simulink model "Scenario_3_v2"  (R2020b)
settings: Solver=ode1be  StartTime=0.0  StopTime=0.5  FixedStep=Ts  MaxStep=Ts/10  MinStep=Ts/40  RelTol=1e-3
values from neighbouring files (symbols this model uses):
  c0 = c0_zeb    (= 6.57988e-09)    [Scenario_17_parameters_v2.m]    (also in Scenario_1_parameters_v2.m; Scenario_2_parameters_v2.m; Scenario_3_parameters_v2.m)
  c0_hawk = 6.37282e-09    [Scenario_17_parameters_v2.m]    (also in Scenario_1_parameters_v2.m; Scenario_2_parameters_v2.m; Scenario_3_parameters_v2.m)
  c1 = c1_zeb    (= 9.15905e-09)    [Scenario_17_parameters_v2.m]    (also in Scenario_1_parameters_v2.m; Scenario_2_parameters_v2.m; Scenario_3_parameters_v2.m)
  c1_hawk = 8.76156e-09    [Scenario_17_parameters_v2.m]    (also in Scenario_1_parameters_v2.m; Scenario_2_parameters_v2.m; Scenario_3_parameters_v2.m)
  fg = 50    [Scenario_17_parameters_v2.m]    (also in Scenario_1_parameters_v2.m; Scenario_2_parameters_v2.m; Scenario_3_parameters_v2.m)
  G10gen = 0.90    (= 0.9)    [Scenario_3_parameters_v2.m]
  G12gen = 0.85    [Scenario_3_parameters_v2.m]
  G1gen = 0.4692    [Scenario_17_parameters_v2.m]    (also in Scenario_1_parameters_v2.m = 0.1; Scenario_2_parameters_v2.m = 0.298581; Scenario_3_parameters_v2.m = 0.65)
  G2gen = 0.80    (= 0.8)    [Scenario_1_parameters_v2.m]    (also in Scenario_2_parameters_v2.m = 0.7; Scenario_3_parameters_v2.m = 0.4)
  G3gen = 0.85    [Scenario_1_parameters_v2.m]    (also in Scenario_2_parameters_v2.m = 0.9; Scenario_3_parameters_v2.m = 0.6)
  G4gen = 0.65    [Scenario_3_parameters_v2.m]
  G5gen = 0.75    [Scenario_17_parameters_v2.m]    (also in Scenario_1_parameters_v2.m = 0.8; Scenario_2_parameters_v2.m = 0.8; Scenario_3_parameters_v2.m = 0.705)
  G6gen = 0.90    (= 0.9)    [Scenario_17_parameters_v2.m]    (also in Scenario_1_parameters_v2.m; Scenario_2_parameters_v2.m = 0.81797; Scenario_3_parameters_v2.m = 0.45)
  G7gen = 0.20    (= 0.2)    [Scenario_17_parameters_v2.m]    (also in Scenario_1_parameters_v2.m = 0.5227; Scenario_2_parameters_v2.m = 0.5098; Scenario_3_parameters_v2.m = 0.4)
  G8gen = 0.58    [Scenario_17_parameters_v2.m]    (also in Scenario_3_parameters_v2.m = 0.65)
  G9gen = 0.8833    [Scenario_17_parameters_v2.m]    (also in Scenario_3_parameters_v2.m = 0.9)
  Iovc = 1.2    [Scenario_17_parameters_v2.m]    (also in Scenario_1_parameters_v2.m; Scenario_2_parameters_v2.m; Scenario_3_parameters_v2.m)
  l0 = l0_zeb    (= 0.00368)    [Scenario_17_parameters_v2.m]    (also in Scenario_1_parameters_v2.m; Scenario_2_parameters_v2.m; Scenario_3_parameters_v2.m)
  l0_hawk = 0.00373    [Scenario_17_parameters_v2.m]    (also in Scenario_1_parameters_v2.m; Scenario_2_parameters_v2.m; Scenario_3_parameters_v2.m)
  l1 = l1_zeb    (= 0.00128)    [Scenario_17_parameters_v2.m]    (also in Scenario_1_parameters_v2.m; Scenario_2_parameters_v2.m; Scenario_3_parameters_v2.m)
  L10dem = 0.04    [Scenario_3_parameters_v2.m]
  L12dem = 0.01    [Scenario_17_parameters_v2.m]    (also in Scenario_3_parameters_v2.m = 0.02)
  L13dem = 0.01    [Scenario_3_parameters_v2.m]
  l1_hawk = 0.00133    [Scenario_17_parameters_v2.m]    (also in Scenario_1_parameters_v2.m; Scenario_2_parameters_v2.m; Scenario_3_parameters_v2.m)
  L1dem = 0.25    [Scenario_17_parameters_v2.m]    (also in Scenario_3_parameters_v2.m = 0.1)
  L3dem = 0.30    (= 0.3)    [Scenario_17_parameters_v2.m]    (also in Scenario_1_parameters_v2.m = 0.1; Scenario_2_parameters_v2.m = 0.1; Scenario_3_parameters_v2.m = 0.2)
  L5dem = 0.25    [Scenario_17_parameters_v2.m]    (also in Scenario_1_parameters_v2.m = 0.35; Scenario_2_parameters_v2.m = 0.35; Scenario_3_parameters_v2.m = 0.1)
  L6dem = 0.15    [Scenario_1_parameters_v2.m]    (also in Scenario_2_parameters_v2.m; Scenario_3_parameters_v2.m = 0.1)
  L7dem = 0.10    (= 0.1)    [Scenario_1_parameters_v2.m]    (also in Scenario_2_parameters_v2.m; Scenario_3_parameters_v2.m = 0.2)
  L9dem = 0.15    [Scenario_17_parameters_v2.m]    (also in Scenario_3_parameters_v2.m = 0.1)
  Pr = Sr*PF    (= 1600500000)    [Scenario_17_parameters_v2.m]    (also in Scenario_1_parameters_v2.m = 1472500000; Scenario_2_parameters_v2.m = 1805000000; Scenario_3_parameters_v2.m = 12740000000)
  Qr = sqrt(Sr^2 - Pr^2)    [Scenario_17_parameters_v2.m]    (also in Scenario_1_parameters_v2.m; Scenario_2_parameters_v2.m; Scenario_3_parameters_v2.m)
  r0 = r0_zeb    (= 0.39362)    [Scenario_17_parameters_v2.m]    (also in Scenario_1_parameters_v2.m; Scenario_2_parameters_v2.m; Scenario_3_parameters_v2.m)
  r0_hawk = 0.44587    [Scenario_17_parameters_v2.m]    (also in Scenario_1_parameters_v2.m; Scenario_2_parameters_v2.m; Scenario_3_parameters_v2.m)
  r1 = r1_zeb    (= 0.06862)    [Scenario_17_parameters_v2.m]    (also in Scenario_1_parameters_v2.m; Scenario_2_parameters_v2.m; Scenario_3_parameters_v2.m)
  r1_hawk = 0.12087    [Scenario_17_parameters_v2.m]    (also in Scenario_1_parameters_v2.m; Scenario_2_parameters_v2.m; Scenario_3_parameters_v2.m)
  Rtpu = Xtpu/40    (= 0.0025)    [Scenario_17_parameters_v2.m]    (also in Scenario_1_parameters_v2.m = 0.00375; Scenario_2_parameters_v2.m = 0.00375; Scenario_3_parameters_v2.m)
  S10non = 500e6    (= 500000000)    [Scenario_3_parameters_v2.m]
  S12non = 250e6    (= 250000000)    [Scenario_3_parameters_v2.m]
  S1non = 700e6    (= 700000000)    [Scenario_17_parameters_v2.m]    (also in Scenario_1_parameters_v2.m = 400000000; Scenario_2_parameters_v2.m = 400000000; Scenario_3_parameters_v2.m = 1000000000)
  S2non = 300e6    (= 300000000)    [Scenario_1_parameters_v2.m]    (also in Scenario_2_parameters_v2.m; Scenario_3_parameters_v2.m = 3000000000)
  S3non = 200e6    (= 200000000)    [Scenario_1_parameters_v2.m]    (also in Scenario_2_parameters_v2.m; Scenario_3_parameters_v2.m = 1000000000)
  S4non = 2000e6    (= 2000000000)    [Scenario_3_parameters_v2.m]
  S5non = 400e6    (= 400000000)    [Scenario_17_parameters_v2.m]    (also in Scenario_1_parameters_v2.m = 500000000; Scenario_2_parameters_v2.m = 500000000; Scenario_3_parameters_v2.m = 2000000000)
  S6non = 150e6    (= 150000000)    [Scenario_17_parameters_v2.m]    (also in Scenario_1_parameters_v2.m = 400000000; Scenario_2_parameters_v2.m = 400000000; Scenario_3_parameters_v2.m = 3000000000)
  S7non = 1500e6    (= 1500000000)    [Scenario_17_parameters_v2.m]    (also in Scenario_1_parameters_v2.m = 200000000; Scenario_2_parameters_v2.m = 200000000; Scenario_3_parameters_v2.m = 4000000000)
  S8non = 600e6    (= 600000000)    [Scenario_17_parameters_v2.m]    (also in Scenario_3_parameters_v2.m = 2000000000)
  S9non = 200e6    (= 200000000)    [Scenario_17_parameters_v2.m]    (also in Scenario_3_parameters_v2.m = 1500000000)
  tonvsc = 0    [Scenario_17_parameters_v2.m]    (also in Scenario_1_parameters_v2.m; Scenario_2_parameters_v2.m; Scenario_3_parameters_v2.m = 0.0001)
  Ts = 50e-6    (= 5e-05)    [Scenario_17_parameters_v2.m]    (also in Scenario_1_parameters_v2.m = 0.0002; Scenario_2_parameters_v2.m = 2e-05; Scenario_3_parameters_v2.m = 0.0001)
  Vhv = 220e3    (= 220000)    [Scenario_17_parameters_v2.m]    (also in Scenario_1_parameters_v2.m; Scenario_2_parameters_v2.m; Scenario_3_parameters_v2.m)
  Vmv = 22e3    (= 22000)    [Scenario_17_parameters_v2.m]    (also in Scenario_1_parameters_v2.m; Scenario_2_parameters_v2.m; Scenario_3_parameters_v2.m)
  w_pll = 2*pi*80    (= 502.654824574)    [Scenario_17_parameters_v2.m]    (also in Scenario_1_parameters_v2.m; Scenario_2_parameters_v2.m; Scenario_3_parameters_v2.m)
  wc1 = wsw1/10    (= 848.230016469)    [Scenario_17_parameters_v2.m]    (also in Scenario_1_parameters_v2.m; Scenario_2_parameters_v2.m; Scenario_3_parameters_v2.m)
  wdc1 = wc1/10    (= 84.8230016469)    [Scenario_17_parameters_v2.m]    (also in Scenario_1_parameters_v2.m; Scenario_2_parameters_v2.m; Scenario_3_parameters_v2.m)
  wpq1 = wc1/10    (= 84.8230016469)    [Scenario_17_parameters_v2.m]    (also in Scenario_1_parameters_v2.m; Scenario_2_parameters_v2.m; Scenario_3_parameters_v2.m)
  wsw1 = ksw1*2*pi*fg    (= 8482.30016469)    [Scenario_17_parameters_v2.m]    (also in Scenario_1_parameters_v2.m; Scenario_2_parameters_v2.m; Scenario_3_parameters_v2.m)
  Xtpu = 0.10    (= 0.1)    [Scenario_17_parameters_v2.m]    (also in Scenario_1_parameters_v2.m = 0.15; Scenario_2_parameters_v2.m = 0.15; Scenario_3_parameters_v2.m)
undefined symbols (not defined in the file or in its folder): D11, Delta
libraries: powerlib x428, simulink_extras x272, powerlib_meascontrol x194, pid_lib x105, simulink x60, eeTransforms x54, spsFirstOrderFilterLib x36, eePwmGeneratorTwoLevel x9
(part 34 of 40)

== system Scenario_3_v2/HVDC/VSC1 v2/VSC Control/Control loops/Phasor PQ 1st/Outer-loop ==
  note: Limits the converter current
  note: Frequency droop
  note: Voltage droop
  note: Reactive power control
  note: Active power control
  note: LVRT
  Pset : Inport
  Qset : Inport  Port=2
  vqd+- : Inport  Port=3
  iqd+- : Inport  Port=4
  freq : Inport  Port=5
  Blk : Inport  Port=6
  Cartesian to Polar : simulink_extras/Transformations/Cartesian to Polar
  Compare To Constant1 : simulink/Logic and Bit Operations/Compare To Constant  relop=<  const=0  OutDataTypeStr=boolean
  Constant1 : Constant  Value=fg
  Constant10 : Constant  Value=0
  Constant11 : Constant  Value=Vlvrt0
  Constant2 : Constant  Value=Vmvpk
  Constant9 : Constant  Value=0
  Demux1 : Demux
  Demux2 : Demux
  Divide1 : Product  Inputs=*/
  Divide2 : Product  Inputs=*/
  First-Order Filter : powerlib_meascontrol/Filters/First-Order Filter  FilterType=Lowpass  Tc=1/wpq  Ts=0  Initialize=on  Vac_Init=[0, 0, 60]  Vdc_Init=Icq  PlotResponse=off  FreqRange="[0,  200,  1]"
  First-Order Filter1 : powerlib_meascontrol/Filters/First-Order Filter  FilterType=Lowpass  Tc=2e-3  Ts=0  Initialize=on  Vac_Init=[0, 0, 60]  Vdc_Init=Vgq  PlotResponse=off  FreqRange="[0,  200,  1]"
  First-Order Filter2 : powerlib_meascontrol/Filters/First-Order Filter  FilterType=Lowpass  Tc=1/wpq  Ts=0  Initialize=on  Vac_Init=[0, 0, 60]  Vdc_Init=Icd  PlotResponse=off  FreqRange="[0,  200,  1]"
  First-Order Filter3 : powerlib_meascontrol/Filters/First-Order Filter  FilterType=Lowpass  Tc=20e-3  Ts=0  Initialize=on  Vac_Init=[0, 0, 60]  Vdc_Init=fg  PlotResponse=off  FreqRange="[0,  200,  1]"
  Gain : Gain  Gain=2/3
  Gain1 : Gain  Gain=2/3
  Gain14 : Gain  Gain=1/Vmvpk
  Gain15 : Gain  Gain=Klvrt
  Gain16 : Gain  Gain=Iconvbase
  Gain5 : Gain  Gain=1/Kfdroop*(Pconv/fg) * fdroop_en
  Gain6 : Gain  Gain=1/Kvdroop*(Pconv/Vmvpk) * Vacdroop_en
  Mux1 : Mux  Inputs=10
  Polar to Cartesian : simulink_extras/Transformations/Polar to Cartesian
      settings: SourceProductBaseCode=SL
  Power calculation : Subsystem
  Saturation : Saturate  UpperLimit=Imax  LowerLimit=0
  Saturation1 : Saturate  UpperLimit=fdroop_per*Pconv  LowerLimit=-fdroop_per*Pconv
  Saturation2 : Saturate  UpperLimit=Vacdroop_per*Pconv  LowerLimit=-Vacdroop_per*Pconv
  Saturation3 : Saturate  UpperLimit=inf  LowerLimit=eps
  Saturation4 : Saturate  UpperLimit=inf  LowerLimit=eps
  Saturation7 : Saturate  UpperLimit=0  LowerLimit=-Qmax_lvrt
  Step : Step  Commented=on  Time=0.1  After=0.3*3711  SampleTime=0
  Step1 : Step  Commented=on  Time=0.2  After=0.2*3711  SampleTime=0
  Sum11 : Sum  Inputs=|+-
  Sum3 : Sum  Inputs=|++
  Sum4 : Sum  Inputs=|+-
  Sum5 : Sum  Inputs=|++
  Sum6 : Sum  Inputs=|+-
  Switch2 : Switch  Threshold=1
  Terminator : Terminator
  iq+* : Outport
  id+* : Outport  Port=2
  iq-* : Outport  Port=3
  id-* : Outport  Port=4
  m : Outport  Port=5
  wires:
  [vqp] -> Saturation4/1
  Saturation4/1 -> Divide2/2
  Divide2/1 -> Gain1/1
  Gain1/1 -> First-Order Filter2/1
  Gain/1 -> First-Order Filter/1
  [vqp] -> Saturation3/1
  Divide1/1 -> Gain/1
  Saturation3/1 -> Divide1/2
  Constant10/1 -> id-*/1
  Constant9/1 -> iq-*/1
  First-Order Filter3/1 -> Sum4/2
  [f] -> First-Order Filter3/1
  Saturation2/1 -> Sum5/2
  Qset/1 -> Sum5/1
  Cartesian to Polar/2 -> Polar to Cartesian/2
  Polar to Cartesian/1 -> iq+*/1
  Polar to Cartesian/2 -> id+*/1
  Cartesian to Polar/1 -> Saturation/1
  Saturation/1 -> Polar to Cartesian/1
  Sum3/1 -> Divide1/1  "Pref"
  Constant1/1 -> Sum4/1
  Sum4/1 -> Gain5/1
  Saturation1/1 -> Sum3/2
  Sum5/1 -> Divide2/1  "Qref"
  Sum6/1 -> Gain6/1
  [vqfilt] -> Sum6/2
  Constant2/1 -> Sum6/1
  Pset/1 -> Sum3/1
  First-Order Filter/1 -> Cartesian to Polar/1
  Blk/1 -> Terminator/1
  freq/1 -> [f]
  [vqp] -> Mux1/1
  Mux1/1 -> m/1
  First-Order Filter1/1 -> [vqfilt]
  vqd+-/1 -> Demux1/1
  iqd+-/1 -> Demux2/1
  Demux1/1 -> First-Order Filter1/1, [vqp]
  Demux1/2 -> [vdp]
  Demux1/3 -> [vqn]
  Demux1/4 -> [vdn]
  Demux2/1 -> [iqp]
  Demux2/2 -> [idp]
  Demux2/3 -> [iqn]
  Demux2/4 -> [idn]
  [vqp] -> Power calculation/1(vq+)
  [iqp] -> Power calculation/3(iq+)
  Power calculation/1(PQ) -> [PQdq]
  [idp] -> Power calculation/4(id+)
  [vdp] -> Power calculation/2(vd+)
  [vqn] -> Power calculation/5(vq-)
  [vdn] -> Power calculation/6(vd-)
  [iqn] -> Power calculation/7(iq-)
  [idn] -> Power calculation/8(id-)
  [LVRT_true] -> Switch2/2
  First-Order Filter2/1 -> Switch2/3
  Switch2/1 -> Cartesian to Polar/2
  Compare To Constant1/1 -> [LVRT_true]
  Gain16/1 -> Switch2/1
  Gain15/1 -> Saturation7/1
  Saturation7/1 -> Compare To Constant1/1, Gain16/1
  [vqfilt] -> Gain14/1
  Sum11/1 -> Gain15/1
  Gain14/1 -> Sum11/2
  Constant11/1 -> Sum11/1
  [vdp] -> Mux1/2
  [vqn] -> Mux1/3
  [vdn] -> Mux1/4
  [iqn] -> Mux1/7
  [idn] -> Mux1/8
  [f] -> Mux1/9
  [PQdq] -> Mux1/10
  [idp] -> Mux1/6
  [iqp] -> Mux1/5
  Gain5/1 -> Saturation1/1
  Gain6/1 -> Saturation2/1

== system Scenario_3_v2/HVDC/VSC1 v2/VSC Control/Control loops/SW, EMT AVG, Phasor Quasi-EMT/Inner-loop ==
  note: Positive-sequence current control
  note: Negative-sequence current control
  iq+* : Inport
  id+* : Inport  Port=2
  iq-* : Inport  Port=3
  id-* : Inport  Port=4
  Blk : Inport  Port=5
  vqd+- : Inport  Port=6
  iqd+- : Inport  Port=7
  Demux1 : Demux
  Demux2 : Demux
  Gain{,1..3} (4 alike) : Gain  Gain=Xt
  NOT{,1..3} (4 alike) : Logic  Operator=NOT  IconShape=distinctive  AllPortsSameDT=off  OutDataTypeStr=boolean
  PID Controller1 : pid_lib/PID Controller  Controller=PI  Form=Ideal  TimeDomain=Continuous-time  UseExternalTs=off  SampleTime=-1  IntegratorMethod=Forward Euler  FilterMethod=Forward Euler  ControllerParametersSource=internal  P=kp_c  I=1/ti_c  D=0  UseFilter=on  N=100  TunerSelectOption=Transfer Function Based (PID Tuner App)  InitialConditionSource=internal  InitialConditionForIntegrator=0  InitialConditionForFilter=0  DifferentiatorICPrevScaledInput=0  ExternalReset=level  TrackingMode=off  Kt=1  LimitOutput=off  SatLimitsSource=internal  UpperSaturationLimit=10*Vmvpk  LowerSaturationLimit=-10*Vmvpk  LinearizeAsGain=off  AntiWindupMode=none  Kb=1  POutMin=[]  POutMax=[]  IOutMin=[]  IOutMax=[]  DOutMin=[]  DOutMax=[]  NOutMin=[]  NOutMax=[]  SumOutMin=[]  SumOutMax=[]  SaturationOutMin=[]  SaturationOutMax=[]  PParamMin=[]  PParamMax=[]  IParamMin=[]  IParamMax=[]  DParamMin=[]  DParamMax=[]  NParamMin=[]  NParamMax=[]  KbParamMin=[]  KbParamMax=[]  KtParamMin=[]  KtParamMax=[]  KbOutMin=[]  KbOutMax=[]  KtOutMin=[]  KtOutMax=[]  IntegratorOutMin=[]  IntegratorOutMax=[]  FilterOutMin=[]  FilterOutMax=[]  SumI1OutMin=[]  SumI1OutMax=[]  SumI2OutMin=[]  SumI2OutMax=[]  SumI3OutMin=[]  SumI3OutMax=[]  SumI4OutMin=[]  SumI4OutMax=[]  SumDOutMin=[]  SumDOutMax=[]  DifferentiatorOutMin=[]  DifferentiatorOutMax=[]  FilterDiffOutCoefMin=[]  FilterDiffOutCoefMax=[]  ReciprocalOutMin=[]  ReciprocalOutMax=[]  SumDenOutMin=[]  SumDenOutMax=[]  SumNumOutMin=[]  SumNumOutMax=[]  DivideOutMin=[]  DivideOutMax=[]  UdiffTsProdOutMin=[]  UdiffTsProdOutMax=[]  NTsProdOutMin=[]  NTsProdOutMax=[]  UintegralTsProdOutMin=[]  UintegralTsProdOutMax=[]  UngainTsProdOutMin=[]  UngainTsProdOutMax=[]  IntegratorContinuousStateAttributes=''  IntegratorStateMustResolveToSignalObject=off  IntegratorRTWStateStorageClass=Auto  FilterContinuousStateAttributes=''  FilterStateMustResolveToSignalObject=off  FilterRTWStateStorageClass=Auto  ParallelPVariant=Passthrough  IdealPVariant=InternalParameters  IVariant=InternalParameters  DVariant=Disabled  IntegratorVariant=Continuous  SatVariant=Disabled  AWVariant=Passthrough  PCopyVariant=Disabled  TRVariant=Disabled  FdbkBlocksVariant=Forward  IdealPFdbkVariant=Disabled  SatFdbkVariant=Disabled  DerivativeFilterVariant=Disabled  NVariant=Disabled  NCopyVariant=Disabled_SignalSpec  FilterICVariant=Disabled  IntegratorICVariant=InternalICs  ExternalResetVariant=ExternalReset  TRSumVariant=Passthrough  SumFdbkVariant=Disabled  SumVariant=Sum_PI  TsampFilterVariant=InternalTs  TsampNgainVariant=Passthrough  TsampIntegralVariant=Passthrough  ExternalSaturationOutDataTypeStr=Inherit: Same as second input
  PID Controller2 : pid_lib/PID Controller  Controller=PI  Form=Ideal  TimeDomain=Continuous-time  UseExternalTs=off  SampleTime=-1  IntegratorMethod=Forward Euler  FilterMethod=Forward Euler  ControllerParametersSource=internal  P=kp_c  I=1/ti_c  D=0  UseFilter=on  N=100  TunerSelectOption=Transfer Function Based (PID Tuner App)  InitialConditionSource=internal  InitialConditionForIntegrator=Tcq/kp_c  InitialConditionForFilter=0  DifferentiatorICPrevScaledInput=0  ExternalReset=level  TrackingMode=off  Kt=1  LimitOutput=off  SatLimitsSource=internal  UpperSaturationLimit=10*Vmvpk  LowerSaturationLimit=-10*Vmvpk  LinearizeAsGain=off  AntiWindupMode=none  Kb=1  POutMin=[]  POutMax=[]  IOutMin=[]  IOutMax=[]  DOutMin=[]  DOutMax=[]  NOutMin=[]  NOutMax=[]  SumOutMin=[]  SumOutMax=[]  SaturationOutMin=[]  SaturationOutMax=[]  PParamMin=[]  PParamMax=[]  IParamMin=[]  IParamMax=[]  DParamMin=[]  DParamMax=[]  NParamMin=[]  NParamMax=[]  KbParamMin=[]  KbParamMax=[]  KtParamMin=[]  KtParamMax=[]  KbOutMin=[]  KbOutMax=[]  KtOutMin=[]  KtOutMax=[]  IntegratorOutMin=[]  IntegratorOutMax=[]  FilterOutMin=[]  FilterOutMax=[]  SumI1OutMin=[]  SumI1OutMax=[]  SumI2OutMin=[]  SumI2OutMax=[]  SumI3OutMin=[]  SumI3OutMax=[]  SumI4OutMin=[]  SumI4OutMax=[]  SumDOutMin=[]  SumDOutMax=[]  DifferentiatorOutMin=[]  DifferentiatorOutMax=[]  FilterDiffOutCoefMin=[]  FilterDiffOutCoefMax=[]  ReciprocalOutMin=[]  ReciprocalOutMax=[]  SumDenOutMin=[]  SumDenOutMax=[]  SumNumOutMin=[]  SumNumOutMax=[]  DivideOutMin=[]  DivideOutMax=[]  UdiffTsProdOutMin=[]  UdiffTsProdOutMax=[]  NTsProdOutMin=[]  NTsProdOutMax=[]  UintegralTsProdOutMin=[]  UintegralTsProdOutMax=[]  UngainTsProdOutMin=[]  UngainTsProdOutMax=[]  IntegratorContinuousStateAttributes=''  IntegratorStateMustResolveToSignalObject=off  IntegratorRTWStateStorageClass=Auto  FilterContinuousStateAttributes=''  FilterStateMustResolveToSignalObject=off  FilterRTWStateStorageClass=Auto  ParallelPVariant=Passthrough  IdealPVariant=InternalParameters  IVariant=InternalParameters  DVariant=Disabled  IntegratorVariant=Continuous  SatVariant=Disabled  AWVariant=Passthrough  PCopyVariant=Disabled  TRVariant=Disabled  FdbkBlocksVariant=Forward  IdealPFdbkVariant=Disabled  SatFdbkVariant=Disabled  DerivativeFilterVariant=Disabled  NVariant=Disabled  NCopyVariant=Disabled_SignalSpec  FilterICVariant=Disabled  IntegratorICVariant=InternalICs  ExternalResetVariant=ExternalReset  TRSumVariant=Passthrough  SumFdbkVariant=Disabled  SumVariant=Sum_PI  TsampFilterVariant=InternalTs  TsampNgainVariant=Passthrough  TsampIntegralVariant=Passthrough  ExternalSaturationOutDataTypeStr=Inherit: Same as second input
  PID Controller3 : pid_lib/PID Controller  Controller=PI  Form=Ideal  TimeDomain=Continuous-time  UseExternalTs=off  SampleTime=-1  IntegratorMethod=Forward Euler  FilterMethod=Forward Euler  ControllerParametersSource=internal  P=kp_c  I=1/ti_c  D=0  UseFilter=on  N=100  TunerSelectOption=Transfer Function Based (PID Tuner App)  InitialConditionSource=internal  InitialConditionForIntegrator=Tcd/kp_c  InitialConditionForFilter=0  DifferentiatorICPrevScaledInput=0  ExternalReset=level  TrackingMode=off  Kt=1  LimitOutput=off  SatLimitsSource=internal  UpperSaturationLimit=10*Vmvpk  LowerSaturationLimit=-10*Vmvpk  LinearizeAsGain=off  AntiWindupMode=none  Kb=1  POutMin=[]  POutMax=[]  IOutMin=[]  IOutMax=[]  DOutMin=[]  DOutMax=[]  NOutMin=[]  NOutMax=[]  SumOutMin=[]  SumOutMax=[]  SaturationOutMin=[]  SaturationOutMax=[]  PParamMin=[]  PParamMax=[]  IParamMin=[]  IParamMax=[]  DParamMin=[]  DParamMax=[]  NParamMin=[]  NParamMax=[]  KbParamMin=[]  KbParamMax=[]  KtParamMin=[]  KtParamMax=[]  KbOutMin=[]  KbOutMax=[]  KtOutMin=[]  KtOutMax=[]  IntegratorOutMin=[]  IntegratorOutMax=[]  FilterOutMin=[]  FilterOutMax=[]  SumI1OutMin=[]  SumI1OutMax=[]  SumI2OutMin=[]  SumI2OutMax=[]  SumI3OutMin=[]  SumI3OutMax=[]  SumI4OutMin=[]  SumI4OutMax=[]  SumDOutMin=[]  SumDOutMax=[]  DifferentiatorOutMin=[]  DifferentiatorOutMax=[]  FilterDiffOutCoefMin=[]  FilterDiffOutCoefMax=[]  ReciprocalOutMin=[]  ReciprocalOutMax=[]  SumDenOutMin=[]  SumDenOutMax=[]  SumNumOutMin=[]  SumNumOutMax=[]  DivideOutMin=[]  DivideOutMax=[]  UdiffTsProdOutMin=[]  UdiffTsProdOutMax=[]  NTsProdOutMin=[]  NTsProdOutMax=[]  UintegralTsProdOutMin=[]  UintegralTsProdOutMax=[]  UngainTsProdOutMin=[]  UngainTsProdOutMax=[]  IntegratorContinuousStateAttributes=''  IntegratorStateMustResolveToSignalObject=off  IntegratorRTWStateStorageClass=Auto  FilterContinuousStateAttributes=''  FilterStateMustResolveToSignalObject=off  FilterRTWStateStorageClass=Auto  ParallelPVariant=Passthrough  IdealPVariant=InternalParameters  IVariant=InternalParameters  DVariant=Disabled  IntegratorVariant=Continuous  SatVariant=Disabled  AWVariant=Passthrough  PCopyVariant=Disabled  TRVariant=Disabled  FdbkBlocksVariant=Forward  IdealPFdbkVariant=Disabled  SatFdbkVariant=Disabled  DerivativeFilterVariant=Disabled  NVariant=Disabled  NCopyVariant=Disabled_SignalSpec  FilterICVariant=Disabled  IntegratorICVariant=InternalICs  ExternalResetVariant=ExternalReset  TRSumVariant=Passthrough  SumFdbkVariant=Disabled  SumVariant=Sum_PI  TsampFilterVariant=InternalTs  TsampNgainVariant=Passthrough  TsampIntegralVariant=Passthrough  ExternalSaturationOutDataTypeStr=Inherit: Same as second input
  PID Controller4 : pid_lib/PID Controller  Controller=PI  Form=Ideal  TimeDomain=Continuous-time  UseExternalTs=off  SampleTime=-1  IntegratorMethod=Forward Euler  FilterMethod=Forward Euler  ControllerParametersSource=internal  P=kp_c  I=1/ti_c  D=0  UseFilter=on  N=100  TunerSelectOption=Transfer Function Based (PID Tuner App)  InitialConditionSource=internal  InitialConditionForIntegrator=0  InitialConditionForFilter=0  DifferentiatorICPrevScaledInput=0  ExternalReset=level  TrackingMode=off  Kt=1  LimitOutput=off  SatLimitsSource=internal  UpperSaturationLimit=10*Vmvpk  LowerSaturationLimit=-10*Vmvpk  LinearizeAsGain=off  AntiWindupMode=none  Kb=1  POutMin=[]  POutMax=[]  IOutMin=[]  IOutMax=[]  DOutMin=[]  DOutMax=[]  NOutMin=[]  NOutMax=[]  SumOutMin=[]  SumOutMax=[]  SaturationOutMin=[]  SaturationOutMax=[]  PParamMin=[]  PParamMax=[]  IParamMin=[]  IParamMax=[]  DParamMin=[]  DParamMax=[]  NParamMin=[]  NParamMax=[]  KbParamMin=[]  KbParamMax=[]  KtParamMin=[]  KtParamMax=[]  KbOutMin=[]  KbOutMax=[]  KtOutMin=[]  KtOutMax=[]  IntegratorOutMin=[]  IntegratorOutMax=[]  FilterOutMin=[]  FilterOutMax=[]  SumI1OutMin=[]  SumI1OutMax=[]  SumI2OutMin=[]  SumI2OutMax=[]  SumI3OutMin=[]  SumI3OutMax=[]  SumI4OutMin=[]  SumI4OutMax=[]  SumDOutMin=[]  SumDOutMax=[]  DifferentiatorOutMin=[]  DifferentiatorOutMax=[]  FilterDiffOutCoefMin=[]  FilterDiffOutCoefMax=[]  ReciprocalOutMin=[]  ReciprocalOutMax=[]  SumDenOutMin=[]  SumDenOutMax=[]  SumNumOutMin=[]  SumNumOutMax=[]  DivideOutMin=[]  DivideOutMax=[]  UdiffTsProdOutMin=[]  UdiffTsProdOutMax=[]  NTsProdOutMin=[]  NTsProdOutMax=[]  UintegralTsProdOutMin=[]  UintegralTsProdOutMax=[]  UngainTsProdOutMin=[]  UngainTsProdOutMax=[]  IntegratorContinuousStateAttributes=''  IntegratorStateMustResolveToSignalObject=off  IntegratorRTWStateStorageClass=Auto  FilterContinuousStateAttributes=''  FilterStateMustResolveToSignalObject=off  FilterRTWStateStorageClass=Auto  ParallelPVariant=Passthrough  IdealPVariant=InternalParameters  IVariant=InternalParameters  DVariant=Disabled  IntegratorVariant=Continuous  SatVariant=Disabled  AWVariant=Passthrough  PCopyVariant=Disabled  TRVariant=Disabled  FdbkBlocksVariant=Forward  IdealPFdbkVariant=Disabled  SatFdbkVariant=Disabled  DerivativeFilterVariant=Disabled  NVariant=Disabled  NCopyVariant=Disabled_SignalSpec  FilterICVariant=Disabled  IntegratorICVariant=InternalICs  ExternalResetVariant=ExternalReset  TRSumVariant=Passthrough  SumFdbkVariant=Disabled  SumVariant=Sum_PI  TsampFilterVariant=InternalTs  TsampNgainVariant=Passthrough  TsampIntegralVariant=Passthrough  ExternalSaturationOutDataTypeStr=Inherit: Same as second input
  Product{,1..3} (4 alike) : Product
  Sum : Sum  Inputs=|+-
  Sum1 : Sum  Inputs=-++
  Sum2 : Sum  Inputs=+++
  Sum3 : Sum  Inputs=-+|
  Sum4 : Sum  Inputs=|+-
  Sum5 : Sum  Inputs=+++
  Sum6 : Sum  Inputs=++-
  Sum7 : Sum  Inputs=-+|
  vq+* : Outport
  vd+* : Outport  Port=2
  vq-* : Outport  Port=3
  vd-* : Outport  Port=4
  wires:
  iq+*/1 -> Sum/1
  [iqp] -> Gain1/1, Sum/2
  [idp] -> Gain/1, Sum3/1
  PID Controller2/1 -> Sum2/2
  Gain/1 -> Sum2/3
  id+*/1 -> Sum3/2
  Blk/1 -> [blk]
  [blk] -> NOT/1, PID Controller2/2
  Product/1 -> PID Controller2/1
  NOT/1 -> Product/2
  [blk] -> PID Controller3/2, NOT1/1
  NOT1/1 -> Product1/2
  Sum3/1 -> Product1/1
  Product1/1 -> PID Controller3/1
  Demux2/2 -> [idp]
  iqd+-/1 -> Demux2/1
  Demux2/4 -> [idn]
  Demux1/3 -> [vqn]
  Demux1/2 -> [vdp]
  Demux1/4 -> [vdn]
  Demux1/1 -> [vqp]
  Demux2/3 -> [iqn]
  Demux2/1 -> [iqp]
  vqd+-/1 -> Demux1/1
  iq-*/1 -> Sum4/1
  [blk] -> PID Controller4/2, NOT3/1
  Sum5/1 -> vd-*/1
  NOT2/1 -> Product2/2
  Sum7/1 -> Product3/1
  id-*/1 -> Sum7/2
  PID Controller4/1 -> Sum5/2
  NOT3/1 -> Product3/2
  Product3/1 -> PID Controller4/1
  PID Controller1/1 -> Sum6/2
  Product2/1 -> PID Controller1/1
  Sum4/1 -> Product2/1
  Gain3/1 -> Sum5/1
  Sum6/1 -> vq-*/1
  [blk] -> NOT2/1, PID Controller1/2
  Gain2/1 -> Sum6/3
  [idn] -> Gain2/1, Sum7/1
  [iqn] -> Gain3/1, Sum4/2
  [vqn] -> Sum6/1
  [vdn] -> Sum5/3
  Sum2/1 -> vq+*/1
  [vqp] -> Sum2/1
  Gain1/1 -> Sum1/1
  Sum1/1 -> vd+*/1
  PID Controller3/1 -> Sum1/2
  [vdp] -> Sum1/3
  Sum/1 -> Product/1

== system Scenario_3_v2/HVDC/VSC1 v2/VSC Control/Control loops/SW, EMT AVG, Phasor Quasi-EMT/Outer-loop ==
  note: DC voltage control
  note: Limits the converter current
  note: Frequency droop
  note: Voltage droop
  note: Reactive power control
  note: Active power control
  note: LVRT
  Pset : Inport
  Qset : Inport  Port=2
  vqd+- : Inport  Port=3
  iqd+- : Inport  Port=4
  freq : Inport  Port=5
  Blk : Inport  Port=6
  Cartesian to Polar : simulink_extras/Transformations/Cartesian to Polar
  Compare To Constant1 : simulink/Logic and Bit Operations/Compare To Constant  relop=<  const=0  OutDataTypeStr=boolean
  Constant : Constant  Value=qmode
  Constant1 : Constant  Value=fg
  Constant10 : Constant  Value=0
  Constant11 : Constant  Value=Vlvrt0
  Constant2 : Constant  Value=Vmvpk
  Constant3 : Constant  Value=dmode
  Constant4 : Constant  Value=0
  Constant9 : Constant  Value=0
  Demux : Demux  Outputs=2
  Demux1 : Demux
  Demux2 : Demux
  Divide : Product  Commented=on  Inputs=**/
  First-Order Filter : powerlib_meascontrol/Filters/First-Order Filter  FilterType=Lowpass  Tc=2e-3  Ts=0  Initialize=on  Vac_Init=[0, 0, 60]  Vdc_Init=Vgq  PlotResponse=off  FreqRange="[0,  200,  1]"
  First-Order Filter1 : powerlib_meascontrol/Filters/First-Order Filter  FilterType=Lowpass  Tc=20e-3  Ts=0  Initialize=on  Vac_Init=[0, 0, 60]  Vdc_Init=fg  PlotResponse=off  FreqRange="[0,  200,  1]"
  From1 : From  Commented=on  GotoTag=Edc
  From3 : From  Commented=on  GotoTag=vq
  From6 : From  Commented=on  GotoTag=Edc
  Gain14 : Gain  Gain=1/Vmvpk
  Gain15 : Gain  Gain=Klvrt
  Gain16 : Gain  Gain=Iconvbase
  Gain3 : Gain  Commented=on  Gain=2/3
  Gain5 : Gain  Gain=1/Kfdroop*(Pconv/fg) * fdroop_en
  Gain6 : Gain  Gain=1/Kvdroop*(Pconv/Vmvpk) * Vacdroop_en
  Mux1 : Mux  Inputs=10
  NOT : Logic  Operator=NOT  IconShape=distinctive  AllPortsSameDT=off  OutDataTypeStr=boolean
  PID Controller1 : pid_lib/PID Controller  Controller=PI  Form=Ideal  TimeDomain=Continuous-time  UseExternalTs=off  SampleTime=-1  IntegratorMethod=Forward Euler  FilterMethod=Forward Euler  ControllerParametersSource=internal  P=kp_pq  I=1/ti_pq  D=0  UseFilter=on  N=100  TunerSelectOption=Transfer Function Based (PID Tuner App)  InitialConditionSource=internal  InitialConditionForIntegrator=Toq/kp_pq  InitialConditionForFilter=0  DifferentiatorICPrevScaledInput=0  ExternalReset=level  TrackingMode=off  Kt=1  LimitOutput=off  SatLimitsSource=internal  UpperSaturationLimit=inf  LowerSaturationLimit=-inf  LinearizeAsGain=on  AntiWindupMode=none  Kb=1  POutMin=[]  POutMax=[]  IOutMin=[]  IOutMax=[]  DOutMin=[]  DOutMax=[]  NOutMin=[]  NOutMax=[]  SumOutMin=[]  SumOutMax=[]  SaturationOutMin=[]  SaturationOutMax=[]  PParamMin=[]  PParamMax=[]  IParamMin=[]  IParamMax=[]  DParamMin=[]  DParamMax=[]  NParamMin=[]  NParamMax=[]  KbParamMin=[]  KbParamMax=[]  KtParamMin=[]  KtParamMax=[]  KbOutMin=[]  KbOutMax=[]  KtOutMin=[]  KtOutMax=[]  IntegratorOutMin=[]  IntegratorOutMax=[]  FilterOutMin=[]  FilterOutMax=[]  SumI1OutMin=[]  SumI1OutMax=[]  SumI2OutMin=[]  SumI2OutMax=[]  SumI3OutMin=[]  SumI3OutMax=[]  SumI4OutMin=[]  SumI4OutMax=[]  SumDOutMin=[]  SumDOutMax=[]  DifferentiatorOutMin=[]  DifferentiatorOutMax=[]  FilterDiffOutCoefMin=[]  FilterDiffOutCoefMax=[]  ReciprocalOutMin=[]  ReciprocalOutMax=[]  SumDenOutMin=[]  SumDenOutMax=[]  SumNumOutMin=[]  SumNumOutMax=[]  DivideOutMin=[]  DivideOutMax=[]  UdiffTsProdOutMin=[]  UdiffTsProdOutMax=[]  NTsProdOutMin=[]  NTsProdOutMax=[]  UintegralTsProdOutMin=[]  UintegralTsProdOutMax=[]  UngainTsProdOutMin=[]  UngainTsProdOutMax=[]  IntegratorContinuousStateAttributes=''  IntegratorStateMustResolveToSignalObject=off  IntegratorRTWStateStorageClass=Auto  FilterContinuousStateAttributes=''  FilterStateMustResolveToSignalObject=off  FilterRTWStateStorageClass=Auto  ParallelPVariant=Passthrough  IdealPVariant=InternalParameters  IVariant=InternalParameters  DVariant=Disabled  IntegratorVariant=Continuous  SatVariant=Disabled  AWVariant=Passthrough  PCopyVariant=Disabled  TRVariant=Disabled  FdbkBlocksVariant=Forward  IdealPFdbkVariant=Disabled  SatFdbkVariant=Disabled  DerivativeFilterVariant=Disabled  NVariant=Disabled  NCopyVariant=Disabled_SignalSpec  FilterICVariant=Disabled  IntegratorICVariant=InternalICs  ExternalResetVariant=ExternalReset  TRSumVariant=Passthrough  SumFdbkVariant=Disabled  SumVariant=Sum_PI  TsampFilterVariant=InternalTs  TsampNgainVariant=Passthrough  TsampIntegralVariant=Passthrough  ExternalSaturationOutDataTypeStr=Inherit: Same as second input
  PID Controller4 : pid_lib/PID Controller  Commented=on  Controller=PI  Form=Ideal  TimeDomain=Continuous-time  UseExternalTs=off  SampleTime=-1  IntegratorMethod=Forward Euler  FilterMethod=Forward Euler  ControllerParametersSource=internal  P=kp_dc  I=ki_dc/kp_dc  D=0  UseFilter=on  N=100  TunerSelectOption=Transfer Function Based (PID Tuner App)  InitialConditionSource=internal  InitialConditionForIntegrator=0  InitialConditionForFilter=0  DifferentiatorICPrevScaledInput=0  ExternalReset=none  TrackingMode=off  Kt=1  LimitOutput=off  SatLimitsSource=internal  UpperSaturationLimit=inf  LowerSaturationLimit=-inf  LinearizeAsGain=on  AntiWindupMode=none  Kb=1  POutMin=[]  POutMax=[]  IOutMin=[]  IOutMax=[]  DOutMin=[]  DOutMax=[]  NOutMin=[]  NOutMax=[]  SumOutMin=[]  SumOutMax=[]  SaturationOutMin=[]  SaturationOutMax=[]  PParamMin=[]  PParamMax=[]  IParamMin=[]  IParamMax=[]  DParamMin=[]  DParamMax=[]  NParamMin=[]  NParamMax=[]  KbParamMin=[]  KbParamMax=[]  KtParamMin=[]  KtParamMax=[]  KbOutMin=[]  KbOutMax=[]  KtOutMin=[]  KtOutMax=[]  IntegratorOutMin=[]  IntegratorOutMax=[]  FilterOutMin=[]  FilterOutMax=[]  SumI1OutMin=[]  SumI1OutMax=[]  SumI2OutMin=[]  SumI2OutMax=[]  SumI3OutMin=[]  SumI3OutMax=[]  SumI4OutMin=[]  SumI4OutMax=[]  SumDOutMin=[]  SumDOutMax=[]  DifferentiatorOutMin=[]  DifferentiatorOutMax=[]  FilterDiffOutCoefMin=[]  FilterDiffOutCoefMax=[]  ReciprocalOutMin=[]  ReciprocalOutMax=[]  SumDenOutMin=[]  SumDenOutMax=[]  SumNumOutMin=[]  SumNumOutMax=[]  DivideOutMin=[]  DivideOutMax=[]  UdiffTsProdOutMin=[]  UdiffTsProdOutMax=[]  NTsProdOutMin=[]  NTsProdOutMax=[]  UintegralTsProdOutMin=[]  UintegralTsProdOutMax=[]  UngainTsProdOutMin=[]  UngainTsProdOutMax=[]  IntegratorContinuousStateAttributes=''  IntegratorStateMustResolveToSignalObject=off  IntegratorRTWStateStorageClass=Auto  FilterContinuousStateAttributes=''  FilterStateMustResolveToSignalObject=off  FilterRTWStateStorageClass=Auto  ParallelPVariant=Passthrough  IdealPVariant=InternalParameters  IVariant=InternalParameters  DVariant=Disabled  IntegratorVariant=Continuous  SatVariant=Disabled  AWVariant=Passthrough  PCopyVariant=Disabled  TRVariant=Disabled  FdbkBlocksVariant=Forward  IdealPFdbkVariant=Disabled  SatFdbkVariant=Disabled  DerivativeFilterVariant=Disabled  NVariant=Disabled  NCopyVariant=Disabled_SignalSpec  FilterICVariant=Disabled  IntegratorICVariant=InternalICs  ExternalResetVariant=Disabled  TRSumVariant=Passthrough  SumFdbkVariant=Disabled  SumVariant=Sum_PI  TsampFilterVariant=InternalTs  TsampNgainVariant=Passthrough  TsampIntegralVariant=Passthrough  ExternalSaturationOutDataTypeStr=Inherit: Same as second input
  PID Controller6 : pid_lib/PID Controller  Controller=PI  Form=Ideal  TimeDomain=Continuous-time  UseExternalTs=off  SampleTime=-1  IntegratorMethod=Forward Euler  FilterMethod=Forward Euler  ControllerParametersSource=internal  P=kp_pq  I=1/ti_pq  D=0  UseFilter=on  N=100  TunerSelectOption=Transfer Function Based (PID Tuner App)  InitialConditionSource=internal  InitialConditionForIntegrator=Tod/kp_pq  InitialConditionForFilter=0  DifferentiatorICPrevScaledInput=0  ExternalReset=level  TrackingMode=off  Kt=1  LimitOutput=off  SatLimitsSource=internal  UpperSaturationLimit=inf  LowerSaturationLimit=-inf  LinearizeAsGain=on  AntiWindupMode=none  Kb=1  POutMin=[]  POutMax=[]  IOutMin=[]  IOutMax=[]  DOutMin=[]  DOutMax=[]  NOutMin=[]  NOutMax=[]  SumOutMin=[]  SumOutMax=[]  SaturationOutMin=[]  SaturationOutMax=[]  PParamMin=[]  PParamMax=[]  IParamMin=[]  IParamMax=[]  DParamMin=[]  DParamMax=[]  NParamMin=[]  NParamMax=[]  KbParamMin=[]  KbParamMax=[]  KtParamMin=[]  KtParamMax=[]  KbOutMin=[]  KbOutMax=[]  KtOutMin=[]  KtOutMax=[]  IntegratorOutMin=[]  IntegratorOutMax=[]  FilterOutMin=[]  FilterOutMax=[]  SumI1OutMin=[]  SumI1OutMax=[]  SumI2OutMin=[]  SumI2OutMax=[]  SumI3OutMin=[]  SumI3OutMax=[]  SumI4OutMin=[]  SumI4OutMax=[]  SumDOutMin=[]  SumDOutMax=[]  DifferentiatorOutMin=[]  DifferentiatorOutMax=[]  FilterDiffOutCoefMin=[]  FilterDiffOutCoefMax=[]  ReciprocalOutMin=[]  ReciprocalOutMax=[]  SumDenOutMin=[]  SumDenOutMax=[]  SumNumOutMin=[]  SumNumOutMax=[]  DivideOutMin=[]  DivideOutMax=[]  UdiffTsProdOutMin=[]  UdiffTsProdOutMax=[]  NTsProdOutMin=[]  NTsProdOutMax=[]  UintegralTsProdOutMin=[]  UintegralTsProdOutMax=[]  UngainTsProdOutMin=[]  UngainTsProdOutMax=[]  IntegratorContinuousStateAttributes=''  IntegratorStateMustResolveToSignalObject=off  IntegratorRTWStateStorageClass=Auto  FilterContinuousStateAttributes=''  FilterStateMustResolveToSignalObject=off  FilterRTWStateStorageClass=Auto  ParallelPVariant=Passthrough  IdealPVariant=InternalParameters  IVariant=InternalParameters  DVariant=Disabled  IntegratorVariant=Continuous  SatVariant=Disabled  AWVariant=Passthrough  PCopyVariant=Disabled  TRVariant=Disabled  FdbkBlocksVariant=Forward  IdealPFdbkVariant=Disabled  SatFdbkVariant=Disabled  DerivativeFilterVariant=Disabled  NVariant=Disabled  NCopyVariant=Disabled_SignalSpec  FilterICVariant=Disabled  IntegratorICVariant=InternalICs  ExternalResetVariant=ExternalReset  TRSumVariant=Passthrough  SumFdbkVariant=Disabled  SumVariant=Sum_PI  TsampFilterVariant=InternalTs  TsampNgainVariant=Passthrough  TsampIntegralVariant=Passthrough  ExternalSaturationOutDataTypeStr=Inherit: Same as second input
  Polar to Cartesian : simulink_extras/Transformations/Polar to Cartesian
      settings: SourceProductBaseCode=SL
  Power calculation : Subsystem
  Product3 : Product
  Saturation : Saturate  UpperLimit=Imax  LowerLimit=0
  Saturation1 : Saturate  UpperLimit=fdroop_per*Pconv  LowerLimit=-fdroop_per*Pconv
  Saturation2 : Saturate  UpperLimit=Vacdroop_per*Pconv  LowerLimit=-Vacdroop_per*Pconv
  Saturation7 : Saturate  UpperLimit=0  LowerLimit=-Qmax_lvrt
  Scope : Scope
  Subsystem2 : Subsystem  mask{Td=10e-3, x0=0}
      mask prompts: Td "Time to hold the initial condition (s)"; x0 "Initial value to hold"
      mask Display: disp('IC')
  Subsystem3 : Subsystem  mask{Td=10e-3, x0=0}
      mask prompts: Td "Time to hold the initial condition (s)"; x0 "Initial value to hold"
      mask Display: disp('IC')
  Sum{,4,6,11} (4 alike) : Sum  Inputs=|+-
  Sum1 : Sum  Commented=on  Inputs=|+-
  Sum2 : Sum  Inputs=-+|
  Sum3 : Sum  Inputs=|++
  Sum5 : Sum  Inputs=|++
  Switch : Switch  Threshold=2
  Switch1 : Switch  Threshold=2
  Switch2 : Switch  Threshold=1
  Vdcref : Constant  Commented=on  Value=Vdc
  iq+* : Outport
  id+* : Outport  Port=2
  iq-* : Outport  Port=3
  id-* : Outport  Port=4
  m : Outport  Port=5
  wires:
  Constant4/1 -> Switch1/1
  Constant10/1 -> id-*/1
  Constant9/1 -> iq-*/1
  [f] -> First-Order Filter1/1
  Saturation2/1 -> Sum5/2
  Qset/1 -> Sum5/1
  Cartesian to Polar/2 -> Polar to Cartesian/2
  Polar to Cartesian/1 -> iq+*/1
  Polar to Cartesian/2 -> id+*/1
  Cartesian to Polar/1 -> Saturation/1
  Saturation/1 -> Polar to Cartesian/1
  PID Controller1/1 -> Scope/1, Switch/3
  Constant/1 -> Switch/2
  Sum1/1 -> PID Controller4/1
  Divide/1 -> Gain3/1
  From1/1 -> Divide/1
  Vdcref/1 -> Sum1/1
  From6/1 -> Sum1/2
  PID Controller4/1 -> Divide/2
  Gain3/1 -> Switch/1
  Sum3/1 -> Sum/1  "Pref"
  Constant1/1 -> Sum4/1
  Gain5/1 -> Saturation1/1
  Sum4/1 -> Gain5/1
  Saturation1/1 -> Sum3/2
  Sum5/1 -> Sum2/2  "Qref"
  Sum6/1 -> Gain6/1
  Gain6/1 -> Saturation2/1
  From3/1 -> Divide/3
  [vqfilt] -> Sum6/2
  Constant2/1 -> Sum6/1
  PID Controller6/1 -> Switch1/3
  Constant3/1 -> Switch1/2
  Pset/1 -> Sum3/1
  Switch/1 -> Cartesian to Polar/1
  Blk/1 -> [blk]
  [vqp] -> Mux1/1
  Mux1/1 -> m/1
  Product3/1 -> PID Controller6/1
  First-Order Filter/1 -> [vqfilt]
  vqd+-/1 -> Demux1/1
  iqd+-/1 -> Demux2/1
  Demux1/1 -> First-Order Filter/1, [vqp]
  Demux1/2 -> [vdp]
  Demux1/3 -> [vqn]
  Demux1/4 -> [vdn]
  Demux2/1 -> [iqp]
  Demux2/2 -> [idp]
  Demux2/3 -> [iqn]
  Demux2/4 -> [idn]
  [vqp] -> Power calculation/1(vq+)
  [iqp] -> Power calculation/3(iq+)
  Power calculation/1(PQ) -> Demux/1, [PQdq]
  [idp] -> Power calculation/4(id+)
  [vdp] -> Power calculation/2(vd+)
  [vqn] -> Power calculation/5(vq-)
  [vdn] -> Power calculation/6(vd-)
  [iqn] -> Power calculation/7(iq-)
  [idn] -> Power calculation/8(id-)
  [LVRT_true] -> NOT/1
  [LVRT_true] -> Switch2/2
  Switch1/1 -> Switch2/3
  Switch2/1 -> Cartesian to Polar/2
  Compare To Constant1/1 -> [LVRT_true]
  Gain15/1 -> Saturation7/1
  Saturation7/1 -> Compare To Constant1/1, Gain16/1
  [vqfilt] -> Gain14/1
  Sum11/1 -> Gain15/1
  Gain14/1 -> Sum11/2
  Constant11/1 -> Sum11/1
  [vdp] -> Mux1/2
  [vqn] -> Mux1/3
  [vdn] -> Mux1/4
  [iqn] -> Mux1/7
  [idn] -> Mux1/8
  [f] -> Mux1/9
  [PQdq] -> Mux1/10
  [idp] -> Mux1/6
  [iqp] -> Mux1/5
  [blk] -> PID Controller1/2
  [blk] -> PID Controller6/2
  Gain16/1 -> Switch2/1
  NOT/1 -> Product3/2
  Demux/1 -> Sum/2  "P"
  Demux/2 -> Sum2/1  "Q"
  Sum/1 -> Subsystem2/1(In1)
  Subsystem2/1(Out1) -> PID Controller1/1
  Sum2/1 -> Subsystem3/1(In1)
  Subsystem3/1(Out1) -> Product3/1
  freq/1 -> [f]
  First-Order Filter1/1 -> Sum4/2

== system Scenario_3_v2/HVDC/VSC1 v2/VSC Control/Measurements/EMT/PLL aligned with positive-sequence ==
  note: PLL
      | aligned with vd+
  Vabc : Inport
  0-vd=-vd : Gain  Gain=-1
  Gain : Gain  Gain=1/(2*pi)
  Integrator : Integrator  InitialCondition=thetaPLL
  Phase-sequence separation : Subsystem
  Subsystem : Subsystem
      mask Display: disp('PI\n')
  Terminator : Terminator
  Terminator1 : Terminator
  Terminator2 : Terminator
  theta : Outport
  f : Outport  Port=2
  wires:
  Integrator/1 -> theta/1, Phase-sequence separation/2(Theta)
  Gain/1 -> f/1
  0-vd=-vd/1 -> Subsystem/1(in)
  Subsystem/1(w) -> Gain/1, Integrator/1
  Vabc/1 -> Phase-sequence separation/1(abc)
  Phase-sequence separation/1(q+) -> Terminator/1
  Phase-sequence separation/2(d+) -> 0-vd=-vd/1  "vd+"
  Phase-sequence separation/3(q-) -> Terminator1/1
  Phase-sequence separation/4(d-) -> Terminator2/1

== system Scenario_3_v2/HVDC/VSC1 v2/VSC Control/Measurements/EMT/Phase-sequence separation2 ==
  note: Phase-sequence separation based on
      | Delayed Signal Cancellation (DSC) method
  abc : Inport
  Theta : Inport  Port=2
  Complex to Real-Imag1 : ComplexToRealImag
  Complex to Real-Imag2 : ComplexToRealImag
  Complex to Real-Imag3 : ComplexToRealImag
  Constant : Constant  Value=negseq_en
  Demux3 : Demux  Outputs=3
  Exp2 : Math  OutputSignalType=complex  SaturateOnIntegerOverflow=on
  Exp3 : Math  OutputSignalType=complex  SaturateOnIntegerOverflow=on
  Gain1 : Gain  Gain=1/2
  Gain4 : Gain  Gain=-1i
  Gain5 : Gain  Gain=1i
  Gain6 : Gain  Gain=1/2
  Gain7 : Gain  Gain=1i
  NOT : Logic  Operator=NOT  IconShape=distinctive  AllPortsSameDT=off  OutDataTypeStr=boolean
  Product3 : Product
  Product4 : Product
  Real-Imag to Complex : RealImagToComplex
  Real-Imag to Complex1 : RealImagToComplex
  Sum1 : Sum  Inputs=|++
  Sum2 : Sum  Inputs=-+|
  Switch : Switch  Criteria=u2 ~= 0
  Terminator3 : Terminator
  Transport Delay2 : TransportDelay  DelayTime=1/4*(1/fg)  BufferSize=1024*4
  Transport Delay3 : TransportDelay  DelayTime=1/4*(1/fg)  BufferSize=1024*4
  abc to Alpha-Beta-Zero : powerlib_meascontrol/Transformations/abc to Alpha-Beta-Zero
  q+ : Outport
  d+ : Outport  Port=2
  q- : Outport  Port=3
  d- : Outport  Port=4
  wires:
  NOT/1 -> Switch/2
  Constant/1 -> NOT/1
  Switch/1 -> Product3/1
  Gain6/1 -> Switch/3
  Sum2/1 -> Gain1/1
  Transport Delay2/1 -> Real-Imag to Complex1/1
  Demux3/1 -> Real-Imag to Complex/1
  Complex to Real-Imag1/2 -> Transport Delay3/1
  Gain1/1 -> Product4/2
  Real-Imag to Complex/1 -> Complex to Real-Imag1/1, Sum2/2, Sum1/1, Switch/1
  Complex to Real-Imag3/1 -> d-/1
  Real-Imag to Complex1/1 -> Gain5/1
  Complex to Real-Imag1/1 -> Transport Delay2/1
  Transport Delay3/1 -> Real-Imag to Complex1/2
  Demux3/2 -> Real-Imag to Complex/2
  Product3/1 -> Complex to Real-Imag2/1
  Product4/1 -> Complex to Real-Imag3/1
  abc to Alpha-Beta-Zero/1 -> Demux3/1
  abc/1 -> abc to Alpha-Beta-Zero/1
  Exp3/1 -> Product4/1
  Complex to Real-Imag3/2 -> q-/1
  Complex to Real-Imag2/2 -> q+/1
  Demux3/3 -> Terminator3/1
  Sum1/1 -> Gain6/1
  Gain5/1 -> Sum2/1, Sum1/2
  Exp2/1 -> Product3/2
  Gain4/1 -> Exp2/1
  Theta/1 -> Gain4/1, Gain7/1
  Gain7/1 -> Exp3/1
  Complex to Real-Imag2/1 -> d+/1

== system Scenario_3_v2/HVDC/VSC1 v2/VSC Control/Measurements/EMT/Phase-sequence separation3 ==
  note: Phase-sequence separation based on
      | Delayed Signal Cancellation (DSC) method
  abc : Inport
  Theta : Inport  Port=2
  Complex to Real-Imag1 : ComplexToRealImag
  Complex to Real-Imag2 : ComplexToRealImag
  Complex to Real-Imag3 : ComplexToRealImag
  Constant : Constant  Value=negseq_en
  Demux3 : Demux  Outputs=3
  Exp2 : Math  OutputSignalType=complex  SaturateOnIntegerOverflow=on
  Exp3 : Math  OutputSignalType=complex  SaturateOnIntegerOverflow=on
  Gain1 : Gain  Gain=1/2
  Gain4 : Gain  Gain=-1i
  Gain5 : Gain  Gain=1i
  Gain6 : Gain  Gain=1/2
  Gain7 : Gain  Gain=1i
  NOT : Logic  Operator=NOT  IconShape=distinctive  AllPortsSameDT=off  OutDataTypeStr=boolean
  Product3 : Product
  Product4 : Product
  Real-Imag to Complex : RealImagToComplex
  Real-Imag to Complex1 : RealImagToComplex
  Sum1 : Sum  Inputs=|++
  Sum2 : Sum  Inputs=-+|
  Switch : Switch  Criteria=u2 ~= 0
  Terminator3 : Terminator
  Transport Delay2 : TransportDelay  DelayTime=1/4*(1/fg)  BufferSize=1024*4
  Transport Delay3 : TransportDelay  DelayTime=1/4*(1/fg)  BufferSize=1024*4
  abc to Alpha-Beta-Zero : powerlib_meascontrol/Transformations/abc to Alpha-Beta-Zero
  q+ : Outport
  d+ : Outport  Port=2
  q- : Outport  Port=3
  d- : Outport  Port=4
  wires:
  Complex to Real-Imag2/1 -> d+/1
  Gain7/1 -> Exp3/1
  Theta/1 -> Gain7/1, Gain4/1
  Gain4/1 -> Exp2/1
  Exp2/1 -> Product3/2
  Gain5/1 -> Sum1/2, Sum2/1
  Sum1/1 -> Gain6/1
  Demux3/3 -> Terminator3/1
  Complex to Real-Imag2/2 -> q+/1
  Complex to Real-Imag3/2 -> q-/1
  Exp3/1 -> Product4/1
  abc/1 -> abc to Alpha-Beta-Zero/1
  abc to Alpha-Beta-Zero/1 -> Demux3/1
  Product4/1 -> Complex to Real-Imag3/1
  Product3/1 -> Complex to Real-Imag2/1
  Demux3/2 -> Real-Imag to Complex/2
  Transport Delay3/1 -> Real-Imag to Complex1/2
  Complex to Real-Imag1/1 -> Transport Delay2/1
  Real-Imag to Complex1/1 -> Gain5/1
  Complex to Real-Imag3/1 -> d-/1
  Real-Imag to Complex/1 -> Switch/1, Sum1/1, Sum2/2, Complex to Real-Imag1/1
  Gain1/1 -> Product4/2
  Complex to Real-Imag1/2 -> Transport Delay3/1
  Demux3/1 -> Real-Imag to Complex/1
  Transport Delay2/1 -> Real-Imag to Complex1/1
  Sum2/1 -> Gain1/1
  Gain6/1 -> Switch/3
  Switch/1 -> Product3/1
  Constant/1 -> NOT/1
  NOT/1 -> Switch/2

== system Scenario_3_v2/HVDC/VSC1 v2/VSC Control/Measurements/Phasor/Frequency (Phasor)1 ==
  note: Calculates the frequency using the derivative of the voltage phase angle
  note: Zero the derivative in the first two time steps to avoid initialization peaks
  note: Avoid numerical peaks
      | Alternative to unwrap function
  Phase : Inport
  Constant : Constant  Value=fg
  Discrete Derivative : simulink/Discrete/Discrete Derivative  gainval=1.0  ICPrevScaledInput=0  OutMin=[]  OutMax=[]  OutDataType=fixdt(1, 16)  OutScaling=2^-10  DoSatur=off
  Gain1 : Gain  Gain=1/(2*pi)
  Product : Product
  Rate Limiter : RateLimiter  RisingSlewLimit=50  FallingSlewLimit=-50  SampleTimeMode=inherited
  Step : Step  Time=2*Ts  SampleTime=0
  Sum : Sum  Inputs=|++
  Freq : Outport
  wires:
  Phase/1 -> Discrete Derivative/1
  Gain1/1 -> Sum/1  "df"
  Constant/1 -> Sum/2
  Sum/1 -> Freq/1
  Step/1 -> Product/1
  Discrete Derivative/1 -> Product/2  "dw"
  Rate Limiter/1 -> Gain1/1
  Product/1 -> Rate Limiter/1
